simulink model "FDIBenchMark"  (Simulink 8.4)
settings: Solver=ode45  StartTime=0.0  StopTime=4400  FixedStep=Ts  RelTol=1e-12
InitFcn:
  | FDIBenchMarkData
values from neighbouring files (symbols this model uses):
  a = 2.2    [FDIBenchMarkData.m]
  Addt = [-(B_dt+B_r)/J_r B_dt/N_g/J_r -K_dt/J_r; eta_dt*B_dt/N_g/J_g -(eta_dt*B_dt/N_g^2+B_g)/J_g eta_dt*K_dt/N_g/J_g; 1 -1/N_g 0]    [FDIBenchMarkData.m]
  Addt2 = [-(B_dt+B_r)/J_r B_dt/N_g/J_r -K_dt/J_r; eta_dt2*B_dt/N_g/J_g -(eta_dt2*B_dt/N_g^2+B_g)/J_g eta_dt2*K_dt/N_g/J_g; 1 -1/N_g 0]    [FDIBenchMarkData.m]
  alpha = 0.1    [FDIBenchMarkData.m]
  alpha_gc = 50    [FDIBenchMarkData.m]
  Bddt = [1/J_r 0; 0 -1/J_g;0 0]    [FDIBenchMarkData.m]
  Bddt2 = [1/J_r 0; 0 -1/J_g;0 0]    [FDIBenchMarkData.m]
  Cddt = [1 0 0;0 1 0]    [FDIBenchMarkData.m]
  Constant_Beta_1_m1 = 5    [FDIBenchMarkData.m]
  Constant_Beta_3_m1 = 10    [FDIBenchMarkData.m]
  Constant_Omega_r_m1 = 1.4    [FDIBenchMarkData.m]
  Constant_tau_gc = 100    [FDIBenchMarkData.m]
  eta_gc = 0.98    [FDIBenchMarkData.m]
  Gain_Beta_2_m2 = 1.2    [FDIBenchMarkData.m]
  Gain_Omega_r_m2 = 1.1    [FDIBenchMarkData.m]
  H = 87    [FDIBenchMarkData.m]
  k = 4.7    [FDIBenchMarkData.m]
  K_i = 1    [FDIBenchMarkData.m]
  K_opt = .5* rho* pi*R^2*eta_dt*R^3*0.4554/(N_g*8)^3    (= 1.21708013189)    [FDIBenchMarkData.m]
  K_p = 4    [FDIBenchMarkData.m]
  L = acker(A', C', vpe)'    [FDIBenchMarkData.m]
  Lungime_Fereastra = 512    [FDIBenchMarkData.m]
  Lungime_Fereastra_2 = 5    [FDIBenchMarkData.m]
  Lungime_Fereastra_3 = 100    [FDIBenchMarkData.m]
  m = 1+alpha*(alpha-1)*R^2/(8*H^2)    (= 0.995085835315)    [FDIBenchMarkData.m]
  m_Beta = 0    [FDIBenchMarkData.m]
  m_omega_g = 0    [FDIBenchMarkData.m]
  m_omega_r = 0    [FDIBenchMarkData.m]
  m_P_g = 0    [FDIBenchMarkData.m]
  m_tau_g = 0    [FDIBenchMarkData.m]
  m_vw = 1.5    [FDIBenchMarkData.m]
  Omega_delta = 15    [FDIBenchMarkData.m]
  omega_n = 11.11    [FDIBenchMarkData.m]
  Omega_nom = 162    [FDIBenchMarkData.m]
  P_r = 4.8e6    (= 4800000)    [FDIBenchMarkData.m]
  R = 57.5    [FDIBenchMarkData.m]
  r = D_rotor/2    (= 57.5)    [FDIBenchMarkData.m]
  r0 = 1.5    [FDIBenchMarkData.m]
  rho = 1.225    [FDIBenchMarkData.m]
  seed = ceil(seed)    [FDIBenchMarkData.m]
  sigma_Beta = 0.2    [FDIBenchMarkData.m]
  sigma_omega_g = 0.05    [FDIBenchMarkData.m]
  sigma_omega_r = 0.004*2*pi    (= 0.0251327412287)    [FDIBenchMarkData.m]
  sigma_P_g = 1e3    (= 1000)    [FDIBenchMarkData.m]
  sigma_tau_g = 90    [FDIBenchMarkData.m]
  sigma_vm = 0.5    [FDIBenchMarkData.m]
  T_sample = 0.05    [FDIBenchMarkData.m]
  Ts = 1/100    (= 0.01)    [FDIBenchMarkData.m]
  turb_int = Turbulence_intensity    (= 12)    [FDIBenchMarkData.m]
  xi = 0.6    [FDIBenchMarkData.m]
undefined symbols (not defined in the file or in its folder): A, Apb, Apb1, Apb2, B, Bpb, Bpb1, Bpb2, C, Cpb, Cpb1, Cpb2, Cq, Fa, Fb, u0
undefined symbols (not defined in the file): turbulence_seeds
(part 2 of 2)

== system FDIBenchMark/Detectie Anomalii/Detectie Fault_3/Ferestruire si Suprapunere Semnal ==
  note: Tipul ferestrei: Dreptunghiulară
      | Lungimea ferestre: Lungime_fereastra
      | Factor de suprapunere: 75%
  Intrare_Semnal : Inport
  Buffer : Buffer  N=Lungime_Fereastra / 4  TreatMby1Signals=One channel
  Delay1 : Delay  DelayLength=Lungime_Fereastra / 4  InitialCondition=0  InputProcessing=Columns as channels (frame based)  SampleTime=Ts
  Delay2 : Delay  DelayLength=Lungime_Fereastra / 4 * 2  InitialCondition=0  InputProcessing=Columns as channels (frame based)  SampleTime=Ts
  Delay3 : Delay  DelayLength=Lungime_Fereastra / 4 * 3  InitialCondition=0  InputProcessing=Columns as channels (frame based)  SampleTime=Ts
  Matrix Concatenate : Concatenate  NumInputs=4  Mode=Multidimensional array
  Zero-Order Hold : ZeroOrderHold  SampleTime=Ts
  Iesire_Semnal : Outport
  wires:
  Delay3/1 -> Matrix Concatenate/1
  Matrix Concatenate/1 -> Iesire_Semnal/1
  Buffer/1 -> Delay2/1, Delay3/1, Matrix Concatenate/4, Delay1/1
  Intrare_Semnal/1 -> Zero-Order Hold/1
  Zero-Order Hold/1 -> Buffer/1
  Delay1/1 -> Matrix Concatenate/3
  Delay2/1 -> Matrix Concatenate/2

== system FDIBenchMark/Detectie Anomalii/Detectie Fault_4/Calcul FFT ==
  Intrare_Semnal : Inport
  MATLAB Function : MATLAB Function  TreatAsAtomicUnit=on  SystemSampleTime=Ts * (Lungime_Fereastra / 4)
  MATLAB Function1 : MATLAB Function  TreatAsAtomicUnit=on  SystemSampleTime=Ts * (Lungime_Fereastra / 4)
  Matrix Concatenate : Concatenate  Mode=Multidimensional array  ConcatenateDimension=2
  Iesire_Matrice : Outport
  wires:
  MATLAB Function1/1(y) -> MATLAB Function/1(u)
  MATLAB Function/1(y_magnitudine) -> Matrix Concatenate/1
  MATLAB Function/2(y_frecventa) -> Matrix Concatenate/2
  Intrare_Semnal/1 -> MATLAB Function1/1(u)
  Matrix Concatenate/1 -> Iesire_Matrice/1

== system FDIBenchMark/Detectie Anomalii/Detectie Fault_4/Calcul Medie ==
  Intrare_Semnal : Inport
  MATLAB Function : MATLAB Function  TreatAsAtomicUnit=on  SystemSampleTime=Ts * Lungime_Fereastra_2
  Iesire_Valoare : Outport
  wires:
  Intrare_Semnal/1 -> MATLAB Function/1(u)
  MATLAB Function/1(y) -> Iesire_Valoare/1

== system FDIBenchMark/Detectie Anomalii/Detectie Fault_4/Decizie Fault_4 ==
  Intrare_Valoare_Medie : Inport
  Intrare_Matrice_FFT : Inport  Port=2
  Delay : Delay  DelayLength=1  InitialCondition=0  SampleTime=Ts * Lungime_Fereastra_2
  Delay1 : Delay  InitialCondition=0  SampleTime=Ts * Lungime_Fereastra_2
  MATLAB Function : MATLAB Function  TreatAsAtomicUnit=on  SystemSampleTime=Ts
  MATLAB Function1 : MATLAB Function  TreatAsAtomicUnit=on  SystemSampleTime=Ts * Lungime_Fereastra_2
  MATLAB Function2 : MATLAB Function  TreatAsAtomicUnit=on  SystemSampleTime=Ts * (Lungime_Fereastra / 4)
  Scope_Decizie_FFT : Scope
      settings: YMin=-0  YMax=2  SaveName=ScopeData3
  Scope_Decizie_Fault_4 : Scope
      settings: SaveName=ScopeData7
  Scope_Decizie_Medie : Scope
      settings: YMin=0  YMax=1  SaveName=ScopeData2
  To Workspace : ToWorkspace  VariableName=Decizie_Medie_Fault_4  SaveFormat=Structure With Time  SampleTime=Ts
  To Workspace1 : ToWorkspace  VariableName=Decizie_FFT_Fault_4  SaveFormat=Structure With Time  SampleTime=Ts
  To Workspace2 : ToWorkspace  VariableName=Decizie_Fault_4  SaveFormat=Structure With Time  SampleTime=Ts
  Iesire_Decizie : Outport
  wires:
  Intrare_Matrice_FFT/1 -> MATLAB Function2/1(u)
  MATLAB Function/1(y) -> Iesire_Decizie/1, To Workspace2/1, Scope_Decizie_Fault_4/1
  MATLAB Function2/1(y) -> To Workspace1/1, Scope_Decizie_FFT/1, MATLAB Function/2(u2)
  Intrare_Valoare_Medie/1 -> Delay1/1, Delay/1, MATLAB Function1/1(u)
  Delay/1 -> MATLAB Function1/2(u1)
  Delay1/1 -> MATLAB Function1/3(u2)
  MATLAB Function1/1(y) -> Scope_Decizie_Medie/1, To Workspace/1, MATLAB Function/1(u1)

== system FDIBenchMark/Detectie Anomalii/Detectie Fault_4/Ferestruire Semnal ==
  note: Tipul ferestrei: Dreptunghiulară
      | Lungimea ferestre: Lungime_fereastra_2
      | Factor de suprapunere: 0%
  Intrare_Semnal : Inport
  Buffer : Buffer  N=Lungime_Fereastra_2  TreatMby1Signals=One channel
  Zero-Order Hold : ZeroOrderHold  SampleTime=Ts
  Iesire_Semnal : Outport
  wires:
  Buffer/1 -> Iesire_Semnal/1
  Intrare_Semnal/1 -> Zero-Order Hold/1
  Zero-Order Hold/1 -> Buffer/1

== system FDIBenchMark/Detectie Anomalii/Detectie Fault_4/Ferestruire si Suprapunere Semnal ==
  note: Tipul ferestrei: Dreptunghiulară
      | Lungimea ferestre: Lungime_fereastra
      | Factor de suprapunere: 75%
  Intrare_Semnal : Inport
  Buffer : Buffer  N=Lungime_Fereastra / 4  TreatMby1Signals=One channel
  Delay1 : Delay  DelayLength=Lungime_Fereastra / 4  InitialCondition=0  InputProcessing=Columns as channels (frame based)  SampleTime=Ts
  Delay2 : Delay  DelayLength=Lungime_Fereastra / 4 * 2  InitialCondition=0  InputProcessing=Columns as channels (frame based)  SampleTime=Ts
  Delay3 : Delay  DelayLength=Lungime_Fereastra / 4 * 3  InitialCondition=0  InputProcessing=Columns as channels (frame based)  SampleTime=Ts
  Matrix Concatenate : Concatenate  NumInputs=4  Mode=Multidimensional array
  Zero-Order Hold : ZeroOrderHold  SampleTime=Ts
  Iesire_Semnal : Outport
  wires:
  Delay3/1 -> Matrix Concatenate/1
  Matrix Concatenate/1 -> Iesire_Semnal/1
  Buffer/1 -> Delay2/1, Delay3/1, Matrix Concatenate/4, Delay1/1
  Intrare_Semnal/1 -> Zero-Order Hold/1
  Zero-Order Hold/1 -> Buffer/1
  Delay1/1 -> Matrix Concatenate/3
  Delay2/1 -> Matrix Concatenate/2

== system FDIBenchMark/Detectie Anomalii/Detectie Fault_5/Calcul Autocorelatie ==
  Intrare_Semnal : Inport
  MATLAB Function : MATLAB Function  TreatAsAtomicUnit=on  SystemSampleTime=Ts * Lungime_Fereastra_3
  Iesire_Vector : Outport
  wires:
  Intrare_Semnal/1 -> MATLAB Function/1(u)
  MATLAB Function/1(y) -> Iesire_Vector/1

== system FDIBenchMark/Detectie Anomalii/Detectie Fault_5/Calcul Autocorelatie1 ==
  Intrare_Semnal : Inport
  MATLAB Function : MATLAB Function  TreatAsAtomicUnit=on  SystemSampleTime=Ts * Lungime_Fereastra_3
  Iesire_Vector : Outport
  wires:
  Intrare_Semnal/1 -> MATLAB Function/1(u)
  MATLAB Function/1(y) -> Iesire_Vector/1

== system FDIBenchMark/Detectie Anomalii/Detectie Fault_5/Calcul Diferenta in Modul ==
  Intrare_Vector_1 : Inport
  Intrare_Vector_2 : Inport  Port=2
  MATLAB Function : MATLAB Function  TreatAsAtomicUnit=on  SystemSampleTime=Ts * Lungime_Fereastra_3
  Iesire_Vector : Outport
  wires:
  Intrare_Vector_1/1 -> MATLAB Function/1(u1)
  MATLAB Function/1(y) -> Iesire_Vector/1
  Intrare_Vector_2/1 -> MATLAB Function/2(u2)

== system FDIBenchMark/Detectie Anomalii/Detectie Fault_5/Calcul Maxim ==
  Intrare_Vector : Inport
  MATLAB Function : MATLAB Function  TreatAsAtomicUnit=on  SystemSampleTime=Ts * Lungime_Fereastra_3
  Iesire_Valoare : Outport
  wires:
  Intrare_Vector/1 -> MATLAB Function/1(u)
  MATLAB Function/1(y) -> Iesire_Valoare/1

== system FDIBenchMark/Detectie Anomalii/Detectie Fault_5/Decizie Fault_5 ==
  Intrare_Valoare_Maxim : Inport
  MATLAB Function : MATLAB Function  TreatAsAtomicUnit=on  SystemSampleTime=Ts
  Scope_Decizie_Fault_5 : Scope
      settings: SaveName=ScopeData7
  To Workspace : ToWorkspace  VariableName=Decizie_Fault_5  SaveFormat=Structure With Time  SampleTime=Ts
  Iesire_Decizie : Outport
  wires:
  MATLAB Function/1(y) -> Iesire_Decizie/1, To Workspace/1, Scope_Decizie_Fault_5/1
  Intrare_Valoare_Maxim/1 -> MATLAB Function/1(u)

== system FDIBenchMark/Detectie Anomalii/Detectie Fault_5/Ferestruire Semnal ==
  note: Tipul ferestrei: Dreptunghiulară
      | Lungimea ferestre: Lungime_fereastra_3
      | Factor de suprapunere: 0%
  Intrare_Semnal : Inport
  Buffer : Buffer  N=Lungime_Fereastra_3  TreatMby1Signals=One channel
  Zero-Order Hold : ZeroOrderHold  SampleTime=Ts
  Iesire_Semnal : Outport
  wires:
  Buffer/1 -> Iesire_Semnal/1
  Intrare_Semnal/1 -> Zero-Order Hold/1
  Zero-Order Hold/1 -> Buffer/1

== system FDIBenchMark/Detectie Anomalii/Detectie Fault_5/Ferestruire Semnal1 ==
  note: Tipul ferestrei: Dreptunghiulară
      | Lungimea ferestre: Lungime_fereastra_3
      | Factor de suprapunere: 0%
  Intrare_Semnal : Inport
  Buffer : Buffer  N=Lungime_Fereastra_3  TreatMby1Signals=One channel
  Zero-Order Hold : ZeroOrderHold  SampleTime=Ts
  Iesire_Semnal : Outport
  wires:
  Buffer/1 -> Iesire_Semnal/1
  Intrare_Semnal/1 -> Zero-Order Hold/1
  Zero-Order Hold/1 -> Buffer/1

== system FDIBenchMark/Detectie Anomalii/Detectie Fault_8/Calcul Reziduu ==
  Intrare_Semnal_Original : Inport
  Intrare_Semnal_Estimat : Inport  Port=2
  MATLAB Function : MATLAB Function  TreatAsAtomicUnit=on  SystemSampleTime=Ts
  Iesire_Reziduu : Outport
  wires:
  Intrare_Semnal_Original/1 -> MATLAB Function/1(u1)
  MATLAB Function/1(y) -> Iesire_Reziduu/1
  Intrare_Semnal_Estimat/1 -> MATLAB Function/2(u2)

== system FDIBenchMark/Detectie Anomalii/Detectie Fault_8/Decizie Fault_8 ==
  Intrare_Reziduu_Filtrat : Inport
  MATLAB Function : MATLAB Function  TreatAsAtomicUnit=on  SystemSampleTime=Ts
  Scope_Decizie_Fault_8 : Scope
      settings: SaveName=ScopeData7
  To Workspace : ToWorkspace  VariableName=Decizie_Fault_8  SaveFormat=Structure With Time  SampleTime=Ts
  Iesire_Decizie : Outport
  wires:
  MATLAB Function/1(y) -> Iesire_Decizie/1, To Workspace/1, Scope_Decizie_Fault_8/1
  Intrare_Reziduu_Filtrat/1 -> MATLAB Function/1(u)

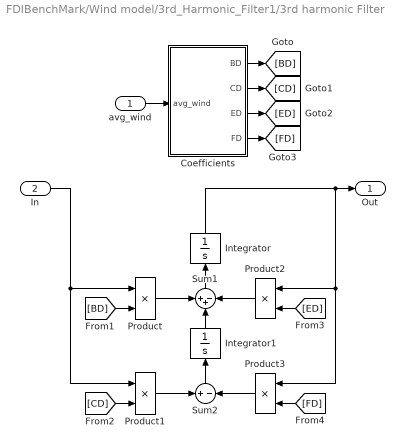
== system FDIBenchMark/Wind model/3rd_Harmonic_Filter1/3rd harmonic Filter ==
  avg_wind : Inport
  In : Inport  Port=2
  Coefficients : Subsystem
  Integrator : Integrator
  Integrator1 : Integrator
  Product{,1..3} (4 alike) : Product  SaturateOnIntegerOverflow=on  OutDataTypeStr=Inherit: Same as first input
  Sum1 : Sum  Inputs=++-  SaturateOnIntegerOverflow=on
  Sum2 : Sum  Inputs=+|-  SaturateOnIntegerOverflow=on
  Out : Outport
  wires:
  avg_wind/1 -> Coefficients/1(avg_wind)
  Coefficients/4(FD) -> [FD]
  Coefficients/3(ED) -> [ED]
  Coefficients/2(CD) -> [CD]
  Coefficients/1(BD) -> [BD]
  [FD] -> Product3/2
  [ED] -> Product2/2
  [CD] -> Product1/2
  [BD] -> Product/2
  In/1 -> Product1/1, Product/1
  Product1/1 -> Sum2/1
  Product3/1 -> Sum2/2
  Sum2/1 -> Integrator1/1
  Product2/1 -> Sum1/3
  Integrator1/1 -> Sum1/2
  Product/1 -> Sum1/1
  Sum1/1 -> Integrator/1
  Integrator/1 -> Out/1, Product3/1, Product2/1

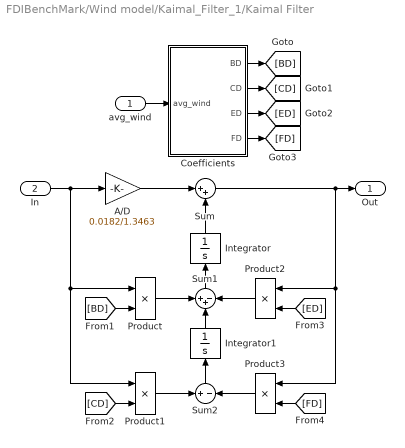
== system FDIBenchMark/Wind model/Kaimal_Filter_1/Kaimal Filter ==
  avg_wind : Inport
  In : Inport  Port=2
  A/D : Gain  Gain=0.0182/1.3463  SaturateOnIntegerOverflow=on  OutDataTypeStr=Inherit: Same as input  ParamDataTypeStr=Inherit: Same as input
  Coefficients : Subsystem
  Integrator : Integrator
  Integrator1 : Integrator
  Product{,1..3} (4 alike) : Product  SaturateOnIntegerOverflow=on  OutDataTypeStr=Inherit: Same as first input
  Sum : Sum  Inputs=|++  SaturateOnIntegerOverflow=on
  Sum1 : Sum  Inputs=++-  SaturateOnIntegerOverflow=on
  Sum2 : Sum  Inputs=+|-  SaturateOnIntegerOverflow=on
  Out : Outport
  wires:
  avg_wind/1 -> Coefficients/1(avg_wind)
  Coefficients/4(FD) -> [FD]
  Coefficients/3(ED) -> [ED]
  Coefficients/2(CD) -> [CD]
  Coefficients/1(BD) -> [BD]
  [FD] -> Product3/2
  [ED] -> Product2/2
  [CD] -> Product1/2
  [BD] -> Product/2
  In/1 -> Product1/1, Product/1, A/D/1
  Sum/1 -> Out/1, Product3/1, Product2/1
  Product1/1 -> Sum2/1
  Product3/1 -> Sum2/2
  Sum2/1 -> Integrator1/1
  Product2/1 -> Sum1/3
  Integrator1/1 -> Sum1/2
  Product/1 -> Sum1/1
  Sum1/1 -> Integrator/1
  Integrator/1 -> Sum/2
  A/D/1 -> Sum/1

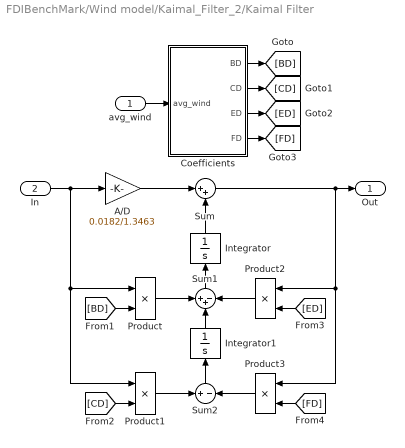
== system FDIBenchMark/Wind model/Kaimal_Filter_2/Kaimal Filter ==
  avg_wind : Inport
  In : Inport  Port=2
  A/D : Gain  Gain=0.0182/1.3463  SaturateOnIntegerOverflow=on  OutDataTypeStr=Inherit: Same as input  ParamDataTypeStr=Inherit: Same as input
  Coefficients : Subsystem
  Integrator : Integrator
  Integrator1 : Integrator
  Product{,1..3} (4 alike) : Product  SaturateOnIntegerOverflow=on  OutDataTypeStr=Inherit: Same as first input
  Sum : Sum  Inputs=|++  SaturateOnIntegerOverflow=on
  Sum1 : Sum  Inputs=++-  SaturateOnIntegerOverflow=on
  Sum2 : Sum  Inputs=+|-  SaturateOnIntegerOverflow=on
  Out : Outport
  wires:
  A/D/1 -> Sum/1
  Integrator/1 -> Sum/2
  Sum1/1 -> Integrator/1
  Product/1 -> Sum1/1
  Integrator1/1 -> Sum1/2
  Product2/1 -> Sum1/3
  Sum2/1 -> Integrator1/1
  Product3/1 -> Sum2/2
  Product1/1 -> Sum2/1
  Sum/1 -> Product2/1, Product3/1, Out/1
  In/1 -> A/D/1, Product/1, Product1/1
  [BD] -> Product/2
  [CD] -> Product1/2
  [ED] -> Product2/2
  [FD] -> Product3/2
  Coefficients/1(BD) -> [BD]
  Coefficients/2(CD) -> [CD]
  Coefficients/3(ED) -> [ED]
  Coefficients/4(FD) -> [FD]
  avg_wind/1 -> Coefficients/1(avg_wind)

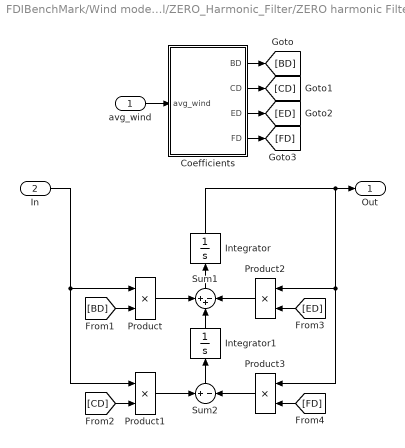
== system FDIBenchMark/Wind model/ZERO_Harmonic_Filter/ZERO harmonic Filter ==
  avg_wind : Inport
  In : Inport  Port=2
  Coefficients : Subsystem
  Integrator : Integrator
  Integrator1 : Integrator
  Product{,1..3} (4 alike) : Product  SaturateOnIntegerOverflow=on  OutDataTypeStr=Inherit: Same as first input
  Sum1 : Sum  Inputs=++-  SaturateOnIntegerOverflow=on
  Sum2 : Sum  Inputs=+|-  SaturateOnIntegerOverflow=on
  Out : Outport
  wires:
  Integrator/1 -> Product2/1, Product3/1, Out/1
  Sum1/1 -> Integrator/1
  Product/1 -> Sum1/1
  Integrator1/1 -> Sum1/2
  Product2/1 -> Sum1/3
  Sum2/1 -> Integrator1/1
  Product3/1 -> Sum2/2
  Product1/1 -> Sum2/1
  In/1 -> Product/1, Product1/1
  [BD] -> Product/2
  [CD] -> Product1/2
  [ED] -> Product2/2
  [FD] -> Product3/2
  Coefficients/1(BD) -> [BD]
  Coefficients/2(CD) -> [CD]
  Coefficients/3(ED) -> [ED]
  Coefficients/4(FD) -> [FD]
  avg_wind/1 -> Coefficients/1(avg_wind)

== system FDIBenchMark/Wind model/3rd_Harmonic_Filter1/3rd harmonic Filter/Coefficients ==
  avg_wind : Inport
  BD coeff : Fcn  Expr=0.2766/0.3691/(r/u(1))
  CD coeff : Fcn  Expr=0.0307/0.3691/(r/u(1))^2
  ED coeff : Fcn  Expr=1.7722/0.3691/(r/u(1))
  FD coeff : Fcn  Expr=1/0.3691/(r/u(1))^2
  BD : Outport
  CD : Outport  Port=2
  ED : Outport  Port=3
  FD : Outport  Port=4
  wires:
  FD coeff/1 -> FD/1
  ED coeff/1 -> ED/1
  CD coeff/1 -> CD/1
  BD coeff/1 -> BD/1
  avg_wind/1 -> FD coeff/1, ED coeff/1, CD coeff/1, BD coeff/1

== system FDIBenchMark/Wind model/Kaimal_Filter_1/Kaimal Filter/Coefficients ==
  avg_wind : Inport
  BD coeff : Fcn  Expr=1.3653/1.3463/(L/2/pi/u(1))
  CD coeff : Fcn  Expr=0.9846/1.3463/(L/2/pi/u(1))^2
  ED coeff : Fcn  Expr=3.7593/1.3463/(L/2/pi/u(1))
  FD coeff : Fcn  Expr=1/1.3463/(L/2/pi/u(1))^2
  BD : Outport
  CD : Outport  Port=2
  ED : Outport  Port=3
  FD : Outport  Port=4
  wires:
  FD coeff/1 -> FD/1
  ED coeff/1 -> ED/1
  CD coeff/1 -> CD/1
  BD coeff/1 -> BD/1
  avg_wind/1 -> FD coeff/1, ED coeff/1, CD coeff/1, BD coeff/1

== system FDIBenchMark/Wind model/Kaimal_Filter_2/Kaimal Filter/Coefficients ==
  avg_wind : Inport
  BD coeff : Fcn  Expr=1.3653/1.3463/(L/2/pi/u(1))
  CD coeff : Fcn  Expr=0.9846/1.3463/(L/2/pi/u(1))^2
  ED coeff : Fcn  Expr=3.7593/1.3463/(L/2/pi/u(1))
  FD coeff : Fcn  Expr=1/1.3463/(L/2/pi/u(1))^2
  BD : Outport
  CD : Outport  Port=2
  ED : Outport  Port=3
  FD : Outport  Port=4
  wires:
  avg_wind/1 -> BD coeff/1, CD coeff/1, ED coeff/1, FD coeff/1
  BD coeff/1 -> BD/1
  CD coeff/1 -> CD/1
  ED coeff/1 -> ED/1
  FD coeff/1 -> FD/1

== system FDIBenchMark/Wind model/ZERO_Harmonic_Filter/ZERO harmonic Filter/Coefficients ==
  avg_wind : Inport
  BD coeff : Fcn  Expr=4.7869/7.6823/(r/u(1))
  CD coeff : Fcn  Expr=0.9904/7.6823/(r/u(1))^2
  ED coeff : Fcn  Expr=7.3518/7.6823/(r/u(1))
  FD coeff : Fcn  Expr=1/7.6823/(r/u(1))^2
  BD : Outport
  CD : Outport  Port=2
  ED : Outport  Port=3
  FD : Outport  Port=4
  wires:
  avg_wind/1 -> BD coeff/1, CD coeff/1, ED coeff/1, FD coeff/1
  BD coeff/1 -> BD/1
  CD coeff/1 -> CD/1
  ED coeff/1 -> ED/1
  FD coeff/1 -> FD/1

== matlab function Detectie Anomalii/Detectie Fault_3/Calcul FFT/MATLAB Function ==
  data: u input double; y_magnitudine output double; y_frecventa output double
function [y_magnitudine, y_frecventa] = Calcul_FFT(u)

    NFFT = 512;
    Ts = 1 / 100;

    X = fft(u, NFFT) / size(u, 1); % calcul FFT
    
    X = X(1 : NFFT / 2 + 1); % retin numai prima jumatate datorita simetriei
    
    y_magnitudine = 2 * abs(X); % calcul magnitudine
    
    y_frecventa = ( (0 : NFFT / 2) * (1 / Ts) / NFFT )'; % calcul frecvente

== matlab function Controller/Embedded MATLAB Function ==
  data: P_g input double; ControlZone output double; P_r input double; Omega_g input double; LastControlZone input double; Omega_nom input double; Omega_delta input double
function ControlZone = ZoneControl(P_g, P_r, Omega_g, LastControlZone,Omega_nom,Omega_delta)
 
if LastControlZone==0,
    if (P_g>=P_r) ||(Omega_g>=Omega_nom)
        ControlZone=1;
    else
        ControlZone=0;
    end
else
    if (Omega_g<(Omega_nom-Omega_delta))
        ControlZone=0;
    else
        ControlZone=1;
    end
end

== matlab function Detectie Anomalii/Detectie Fault_3/Calcul FFT/MATLAB Function1 ==
  data: u input double; y output double
function y = Aplicare_Functie_Fereastra(u)

    Lungime_Fereastra = 512;

    w = hann(Lungime_Fereastra);
    
    y = u .* w;

== matlab function Detectie Anomalii/Detectie Fault_3/Calcul Medie/MATLAB Function ==
  data: u input double; y output double
function y = Calcul_Medie(u)

    y = mean(u);

== matlab function Detectie Anomalii/Detectie Fault_3/Decizie Fault_3/MATLAB Function ==
  data: u1 input double; y output double; u2 input double
function y = Decizie_Fault_3(u1, u2)

    if (u1 == 1 && u2 == 1)
        y = 2; % stare critica 
    else
        if (u1 == 1 || u2 == 1)
            y = 1; % stare de avertizare
        else
            y = 0; % functionare normala
        end;
    end;

== matlab function Detectie Anomalii/Detectie Fault_3/Decizie Fault_3/MATLAB Function1 ==
  data: u input double; u1 input double; y output double; u2 input double
function y = Decizie_Medie(u, u1, u2)

    if (u == u1 && u1 == u2)
        y = 1; % anomalie
    else
        y = 0; % nu a intervenit anomalia
    end;

== matlab function Detectie Anomalii/Detectie Fault_3/Decizie Fault_3/MATLAB Function2 ==
  data: u input double; y output double
function y = Decizie_FFT(u)
  
    NFFT = 512;

    [max_magnitudine, index_max_magnitudine] = max( u(:, 1) );
    
    if ( index_max_magnitudine == 1 && sum( u(4 : NFFT / 2 + 1) ) < 0.01  )
        y = 1; % anomalie
    else
        y = 0; % nu a intervenit anomalia
    end;

== matlab function Detectie Anomalii/Detectie Fault_4/Calcul FFT/MATLAB Function ==
  data: u input double; y_magnitudine output double; y_frecventa output double
function [y_magnitudine, y_frecventa] = Calcul_FFT(u)

    NFFT = 512;
    Ts = 1 / 100;

    X = fft(u, NFFT) / size(u, 1); % calcul FFT
    
    X = X(1 : NFFT / 2 + 1); % retin numai prima jumatate datorita simetriei
    
    y_magnitudine = 2 * abs(X); % calcul magnitudine
    
    y_frecventa = ( (0 : NFFT / 2) * (1 / Ts) / NFFT )'; % calcul frecvente

== matlab function Detectie Anomalii/Detectie Fault_4/Calcul FFT/MATLAB Function1 ==
  data: u input double; y output double
function y = Aplicare_Functie_Fereastra(u)

    Lungime_Fereastra = 512;

    w = hann(Lungime_Fereastra);
    
    y = u .* w;

== matlab function Detectie Anomalii/Detectie Fault_4/Calcul Medie/MATLAB Function ==
  data: u input double; y output double
function y = Calcul_Medie(u)

    y = mean(u);

== matlab function Detectie Anomalii/Detectie Fault_4/Decizie Fault_4/MATLAB Function ==
  data: u1 input double; y output double; u2 input double
function y = Decizie_Fault_4(u1, u2)

    if (u1 == 1 && u2 == 1)
        y = 2; % stare critica 
    else
        if (u1 == 1 || u2 == 1)
            y = 1; % stare de avertizare
        else
            y = 0; % functionare normala
        end;
    end;

== matlab function Detectie Anomalii/Detectie Fault_1/Calcul Medie/MATLAB Function ==
  data: u input double; y output double
function y = Calcul_Medie(u)

    y = mean(u)

== matlab function Detectie Anomalii/Detectie Fault_1/Decizie Fault_1/MATLAB Function ==
  data: u1 input double; y output double; u2 input double
function y = Decizie_Fault_1(u1, u2)

    if (u1 == 1 && u2 == 1)
        y = 2; % stare critica 
    else
        if (u1 == 1 || u2 == 1)
            y = 1; % stare de avertizare
        else
            y = 0; % functionare normala
        end;
    end;

== matlab function Detectie Anomalii/Detectie Fault_1/Calcul FFT/MATLAB Function ==
  data: u input double; y_magnitudine output double; y_frecventa output double
function [y_magnitudine, y_frecventa] = Calcul_FFT(u)

    NFFT = 512;
    Ts = 1 / 100;

    X = fft(u, NFFT) / size(u, 1); % calcul FFT
    
    X = X(1 : NFFT / 2 + 1); % retin numai prima jumatate datorita simetriei
    
    y_magnitudine = 2 * abs(X); % calcul magnitudine
    
    y_frecventa = ( (0 : NFFT / 2) * (1 / Ts) / NFFT )'; % calcul frecvente

== matlab function Detectie Anomalii/Detectie Fault_1/Calcul FFT/MATLAB Function1 ==
  data: u input double; y output double
function y = Aplicare_Functie_Fereastra(u)

    Lungime_Fereastra = 512;

    w = hann(Lungime_Fereastra);
    
    y = u .* w;

== matlab function Detectie Anomalii/Detectie Fault_1/Decizie Fault_1/MATLAB Function1 ==
  data: u input double; u1 input double; y output double; u2 input double
function y = Decizie_Medie(u, u1, u2)

    if (u == u1 && u1 == u2)
        y = 1; % anomalie
    else
        y = 0; % nu a intervenit anomalia
    end;

== matlab function Detectie Anomalii/Detectie Fault_1/Decizie Fault_1/MATLAB Function2 ==
  data: u input double; y output double
function y = Decizie_FFT(u)
  
    NFFT = 512;

    [max_magnitudine, index_max_magnitudine] = max( u(:, 1) );
    
    if ( index_max_magnitudine == 1 && sum( u(4 : NFFT / 2 + 1) ) < 0.01  )
        y = 1; % anomalie
    else
        y = 0; % nu a intervenit anomalia
    end;

== matlab function Detectie Anomalii/Detectie Fault_4/Decizie Fault_4/MATLAB Function1 ==
  data: u input double; u1 input double; y output double; u2 input double
function y = Decizie_Medie(u, u1, u2)

    if (u == u1 && u1 == u2)
        y = 1; % anomalie
    else
        y = 0; % nu a intervenit anomalia
    end;

== matlab function Detectie Anomalii/Detectie Fault_4/Decizie Fault_4/MATLAB Function2 ==
  data: u input double; y output double
function y = Decizie_FFT(u)
  
    NFFT = 512;

    [max_magnitudine, index_max_magnitudine] = max( u(:, 1) );
    
    if ( index_max_magnitudine == 1 && sum( u(4 : NFFT / 2 + 1) ) < 0.01  )
        y = 1; % anomalie
    else
        y = 0; % nu a intervenit anomalia
    end;

== matlab function Detectie Anomalii/Detectie Fault_5/Calcul Autocorelatie/MATLAB Function ==
  data: u input double; y output double
function y = Calcul_Autocorelatie(u)

    y = xcorr(u);

== matlab function Detectie Anomalii/Detectie Fault_5/Calcul Autocorelatie1/MATLAB Function ==
  data: u input double; y output double
function y = Calcul_Autocorelatie(u)

    y = xcorr(u);

== matlab function Detectie Anomalii/Detectie Fault_5/Calcul Diferenta in Modul/MATLAB Function ==
  data: u1 input double; y output double; u2 input double
function y = Calcul_Diferenta_in_Modul(u1, u2)

    y = abs(u1 - u2);

== matlab function Detectie Anomalii/Detectie Fault_5/Calcul Maxim/MATLAB Function ==
  data: u input double; y output double
function y = Calcul_Maxim(u)

    y = max(u);

== matlab function Detectie Anomalii/Detectie Fault_5/Decizie Fault_5/MATLAB Function ==
  data: u input double; y output double
function y = Decizie_Fault_5(u)

    prag = 3 * 10 ^ 4;

    if (u >= prag)
        y = 2; % stare critica
    else
        y = 0; % functionare normala
    end;

== matlab function Detectie Anomalii/Detectie Fault_8/Decizie Fault_8/MATLAB Function ==
  data: u input double; y output double
function y = Decizie_Fault_8(u)

    prag = 30;

    if (u >= prag)
        y = 2; % stare critica
    else
        y = 0; % functionare normala
    end;

== matlab function Detectie Anomalii/Detectie Fault_8/Calcul Reziduu/MATLAB Function ==
  data: u1 input double; y output double; u2 input double
function y = Calcul_Reziduu(u1, u2)

    y = u1 - u2;
